simulink library "PAYLOAD_MASTER"  (Simulink 8.8)
settings: Solver=ode45  StartTime=0.0  StopTime=10.0  RelTol=1e-3  EnableMultiTasking=on
libraries: cdsEpicsOut x123, cdsFilt x55, cdsTP x42, cdsFiltCtrl x33, cdsEpicsIn x31, cdsMuxMatrix x17, cdsEpicsBinIn x17, VIS_LIB x13, PAYLOAD_MASTER x13, cdsRms x8, simulink x6, cdsEpicsStringIn x6
(part 12 of 12)

== system PAYLOAD_MASTER/PAYLOADWD/OPLEVAC ==
  TILT_SEG1_In : Inport
  TILT_SEG2_In : Inport  Port=2
  TILT_SEG3_In : Inport  Port=3
  TILT_SEG4_In : Inport  Port=4
  LEN_SEG1_In : Inport  Port=5
  LEN_SEG2_In : Inport  Port=6
  LEN_SEG3_In : Inport  Port=7
  LEN_SEG4_In : Inport  Port=8
  BANDLIM : Subsystem
  LEN_SEG1RMS : cdsRms/Subsystem  Tag=cdsRms  Description=|
      | Purpose:
      | Calculate an RMS based on the input signal.
      settings: AttributesFormatString=%<Tag>
  LEN_SEG1_RMS : cdsTP/Subsystem  Tag=Test Point
      settings: AttributesFormatString=%<Tag>
  LEN_SEG1_RMSMON : cdsEpicsOut/Subsystem  Tag=cdsEpicsOutput  Description=|
      | Purpose:                                          
      | Output a FE signal to an EPICS channel.           
      |                                                   
      | Operation:                                        
      | Takes input value and passes it to EPICS record.  
      |                                                   
      | Usage:                                            
      | Name the part with the desired EPICS rrecord name.
      settings: AttributesFormatString=%<Tag>
  LEN_SEG2RMS : cdsRms/Subsystem  Tag=cdsRms  Description=|
      | Purpose:
      | Calculate an RMS based on the input signal.
      settings: AttributesFormatString=%<Tag>
  LEN_SEG2_RMS : cdsTP/Subsystem  Tag=Test Point
      settings: AttributesFormatString=%<Tag>
  LEN_SEG2_RMSMON : cdsEpicsOut/Subsystem  Tag=cdsEpicsOutput  Description=|
      | Purpose:                                          
      | Output a FE signal to an EPICS channel.           
      |                                                   
      | Operation:                                        
      | Takes input value and passes it to EPICS record.  
      |                                                   
      | Usage:                                            
      | Name the part with the desired EPICS rrecord name.
      settings: AttributesFormatString=%<Tag>
  LEN_SEG3RMS : cdsRms/Subsystem  Tag=cdsRms  Description=|
      | Purpose:
      | Calculate an RMS based on the input signal.
      settings: AttributesFormatString=%<Tag>
  LEN_SEG3_RMS : cdsTP/Subsystem  Tag=Test Point
      settings: AttributesFormatString=%<Tag>
  LEN_SEG3_RMSMON : cdsEpicsOut/Subsystem  Tag=cdsEpicsOutput  Description=|
      | Purpose:                                          
      | Output a FE signal to an EPICS channel.           
      |                                                   
      | Operation:                                        
      | Takes input value and passes it to EPICS record.  
      |                                                   
      | Usage:                                            
      | Name the part with the desired EPICS rrecord name.
      settings: AttributesFormatString=%<Tag>
  LEN_SEG4RMS : cdsRms/Subsystem  Tag=cdsRms  Description=|
      | Purpose:
      | Calculate an RMS based on the input signal.
      settings: AttributesFormatString=%<Tag>
  LEN_SEG4_RMS : cdsTP/Subsystem  Tag=Test Point
      settings: AttributesFormatString=%<Tag>
  LEN_SEG4_RMSMON : cdsEpicsOut/Subsystem  Tag=cdsEpicsOutput  Description=|
      | Purpose:                                          
      | Output a FE signal to an EPICS channel.           
      |                                                   
      | Operation:                                        
      | Takes input value and passes it to EPICS record.  
      |                                                   
      | Usage:                                            
      | Name the part with the desired EPICS rrecord name.
      settings: AttributesFormatString=%<Tag>
  Operator{1,3..8} (7 alike) : RelationalOperator  Operator=>  OutDataTypeStr=boolean  RndMeth=Nearest
  Operator2 : RelationalOperator  Operator=>  OutDataTypeStr=boolean  ZeroCross=off  RndMeth=Nearest
  RMS_MAX : cdsEpicsIn/Subsystem  Tag=cdsEpicsIn  Description=|
      | Purpose:                                                                              
      | Create an EPICS input channel connection to the FE realtime controls.                 
      |                                                                                       
      | Operation:                                                                            
      | Outputs value from an EPICS ai record. Value is floating point with a precision of 3..
      |                                                                                       
      | Usage:                                                                                
      | Name the part with the desired EPICS channel name.
      settings: AttributesFormatString=%<Tag>
  Sum1 : Sum  Inputs=++++++++
  TILT_SEG1RMS : cdsRms/Subsystem  Tag=cdsRms  Description=|
      | Purpose:
      | Calculate an RMS based on the input signal.
      settings: AttributesFormatString=%<Tag>
  TILT_SEG1_RMS : cdsTP/Subsystem  Tag=Test Point
      settings: AttributesFormatString=%<Tag>
  TILT_SEG1_RMSMON : cdsEpicsOut/Subsystem  Tag=cdsEpicsOutput  Description=|
      | Purpose:                                          
      | Output a FE signal to an EPICS channel.           
      |                                                   
      | Operation:                                        
      | Takes input value and passes it to EPICS record.  
      |                                                   
      | Usage:                                            
      | Name the part with the desired EPICS rrecord name.
      settings: AttributesFormatString=%<Tag>
  TILT_SEG2RMS : cdsRms/Subsystem  Tag=cdsRms  Description=|
      | Purpose:
      | Calculate an RMS based on the input signal.
      settings: AttributesFormatString=%<Tag>
  TILT_SEG2_RMS : cdsTP/Subsystem  Tag=Test Point
      settings: AttributesFormatString=%<Tag>
  TILT_SEG2_RMSMON : cdsEpicsOut/Subsystem  Tag=cdsEpicsOutput  Description=|
      | Purpose:                                          
      | Output a FE signal to an EPICS channel.           
      |                                                   
      | Operation:                                        
      | Takes input value and passes it to EPICS record.  
      |                                                   
      | Usage:                                            
      | Name the part with the desired EPICS rrecord name.
      settings: AttributesFormatString=%<Tag>
  TILT_SEG3RMS : cdsRms/Subsystem  Tag=cdsRms  Description=|
      | Purpose:
      | Calculate an RMS based on the input signal.
      settings: AttributesFormatString=%<Tag>
  TILT_SEG3_RMS : cdsTP/Subsystem  Tag=Test Point
      settings: AttributesFormatString=%<Tag>
  TILT_SEG3_RMSMON : cdsEpicsOut/Subsystem  Tag=cdsEpicsOutput  Description=|
      | Purpose:                                          
      | Output a FE signal to an EPICS channel.           
      |                                                   
      | Operation:                                        
      | Takes input value and passes it to EPICS record.  
      |                                                   
      | Usage:                                            
      | Name the part with the desired EPICS rrecord name.
      settings: AttributesFormatString=%<Tag>
  TILT_SEG4RMS : cdsRms/Subsystem  Tag=cdsRms  Description=|
      | Purpose:
      | Calculate an RMS based on the input signal.
      settings: AttributesFormatString=%<Tag>
  TILT_SEG4_RMS : cdsTP/Subsystem  Tag=Test Point
      settings: AttributesFormatString=%<Tag>
  TILT_SEG4_RMSMON : cdsEpicsOut/Subsystem  Tag=cdsEpicsOutput  Description=|
      | Purpose:                                          
      | Output a FE signal to an EPICS channel.           
      |                                                   
      | Operation:                                        
      | Takes input value and passes it to EPICS record.  
      |                                                   
      | Usage:                                            
      | Name the part with the desired EPICS rrecord name.
      settings: AttributesFormatString=%<Tag>
  FLAG : Outport
  wires:
  TILT_SEG3_RMSMON/1 -> Operator3/1
  TILT_SEG2_RMSMON/1 -> Operator2/1
  TILT_SEG1_RMSMON/1 -> Operator1/1
  Sum1/1 -> FLAG/1
  TILT_SEG3RMS/1 -> TILT_SEG3_RMSMON/1, TILT_SEG3_RMS/1
  TILT_SEG1RMS/1 -> TILT_SEG1_RMSMON/1, TILT_SEG1_RMS/1
  TILT_SEG2RMS/1 -> TILT_SEG2_RMSMON/1, TILT_SEG2_RMS/1
  Operator3/1 -> Sum1/3
  Operator2/1 -> Sum1/2
  Operator1/1 -> Sum1/1
  TILT_SEG1_In/1 -> BANDLIM/1(TILT_SEG1_In)
  TILT_SEG2_In/1 -> BANDLIM/2(TILT_SEG2_In)
  TILT_SEG3_In/1 -> BANDLIM/3(TILT_SEG3_In)
  BANDLIM/1(TILT_SEG1_Out) -> TILT_SEG1RMS/1
  BANDLIM/2(TILT_SEG2_Out) -> TILT_SEG2RMS/1
  BANDLIM/3(TILT_SEG3_Out) -> TILT_SEG3RMS/1
  TILT_SEG4_In/1 -> BANDLIM/4(TILT_SEG4_In)
  LEN_SEG1_In/1 -> BANDLIM/5(LEN_SEG1_In)
  LEN_SEG2_In/1 -> BANDLIM/6(LEN_SEG2_In)
  LEN_SEG3_In/1 -> BANDLIM/7(LEN_SEG3_In)
  LEN_SEG4_In/1 -> BANDLIM/8(LEN_SEG4_In)
  TILT_SEG4RMS/1 -> TILT_SEG4_RMSMON/1, TILT_SEG4_RMS/1
  LEN_SEG1RMS/1 -> LEN_SEG1_RMSMON/1, LEN_SEG1_RMS/1
  LEN_SEG2RMS/1 -> LEN_SEG2_RMSMON/1, LEN_SEG2_RMS/1
  LEN_SEG3RMS/1 -> LEN_SEG3_RMSMON/1, LEN_SEG3_RMS/1
  LEN_SEG4RMS/1 -> LEN_SEG4_RMSMON/1, LEN_SEG4_RMS/1
  BANDLIM/4(TILT_SEG4_Out) -> TILT_SEG4RMS/1
  BANDLIM/5(LEN_SEG1_Out) -> LEN_SEG1RMS/1
  BANDLIM/6(LEN_SEG2_Out) -> LEN_SEG2RMS/1
  BANDLIM/7(LEN_SEG3_Out) -> LEN_SEG3RMS/1
  BANDLIM/8(LEN_SEG4_Out) -> LEN_SEG4RMS/1
  TILT_SEG4_RMSMON/1 -> Operator4/1
  LEN_SEG1_RMSMON/1 -> Operator5/1
  LEN_SEG2_RMSMON/1 -> Operator7/1
  LEN_SEG3_RMSMON/1 -> Operator6/1
  LEN_SEG4_RMSMON/1 -> Operator8/1
  RMS_MAX/1 -> Operator8/2, Operator6/2, Operator7/2, Operator5/2, Operator4/2, Operator3/2, Operator2/2, Operator1/2
  Operator4/1 -> Sum1/4
  Operator5/1 -> Sum1/5
  Operator7/1 -> Sum1/6
  Operator6/1 -> Sum1/7
  Operator8/1 -> Sum1/8

== system PAYLOAD_MASTER/PAYLOAD_MASTER/BIO ==
  note: 12 Bit Word
  note: 12 Bit Word
  TM_ISC_CTRL : Inport
  TM_MON_In : Inport  Port=2
  IM1_CTRL : Inport  Port=3
  IM1_MON_In : Inport  Port=4
  IM2_ISC_CTRL : Inport  Port=5
  IM2_MON_In : Inport  Port=6
  IM1 : STATE_BIO_MASTER/UIM_BIO_MASTER
  IM2 : STATE_BIO_MASTER/UIM_BIO_MASTER
  TM : STATE_BIO_MASTER/UIM_BIO_MASTER
  TM_BO_CTRL_Out : Outport
  TM_MASK_Out : Outport  Port=2
  TM_CTRL_Out : Outport  Port=3
  IM1_BO_CTRL_Out : Outport  Port=4
  IM1_MASK_Out : Outport  Port=5
  IM1_CTRL_Out : Outport  Port=6
  IM2_BO_CTRL_Out : Outport  Port=7
  IM2_MASK_Out : Outport  Port=8
  IM2_CTRL_Out : Outport  Port=9
  wires:
  IM2/3 -> IM2_BO_CTRL_Out/1
  IM2/2 -> IM2_CTRL_Out/1
  IM2/1 -> IM2_MASK_Out/1
  IM1/3 -> IM1_BO_CTRL_Out/1
  IM1/2 -> IM1_CTRL_Out/1
  IM1/1 -> IM1_MASK_Out/1
  TM/3 -> TM_BO_CTRL_Out/1
  TM/2 -> TM_CTRL_Out/1
  TM/1 -> TM_MASK_Out/1
  IM2_ISC_CTRL/1 -> IM2/1
  IM2_MON_In/1 -> IM2/2
  IM1_MON_In/1 -> IM1/2
  IM1_CTRL/1 -> IM1/1
  TM_ISC_CTRL/1 -> TM/1
  TM_MON_In/1 -> TM/2

== system PAYLOAD_MASTER/PAYLOADWD/OPLEVAC/BANDLIM ==
  TILT_SEG1_In : Inport
  TILT_SEG2_In : Inport  Port=2
  TILT_SEG3_In : Inport  Port=3
  TILT_SEG4_In : Inport  Port=4
  LEN_SEG1_In : Inport  Port=5
  LEN_SEG2_In : Inport  Port=6
  LEN_SEG3_In : Inport  Port=7
  LEN_SEG4_In : Inport  Port=8
  LEN_SEG1 : cdsFilt/Subsystem  Tag=cdsFilt  Description=|
      | Purpose:                                                                                                                                                                                                                                  
      | Standard CDS IIR filter module.                                                                                                                                                                                                           
      |                                                                                                                                                                                                                                           
      | Operation:                                                                                                                                                                                                                                
      | Consists of 10 second order section IIR filters, plus a ramped gain stage. In FE code, also provides pre-defined test points and excitation channel inputs. The filter coefficients are defined in the LIGO system using the 'foton' tool.
      |                                                                                                                                                                                                                                           
      | Usage:                                                                                                                                                                                                                                    
      | Name the part with the desired filter module name.
      settings: AttributesFormatString=%<Tag>
  LEN_SEG2 : cdsFilt/Subsystem  Tag=cdsFilt  Description=|
      | Purpose:                                                                                                                                                                                                                                  
      | Standard CDS IIR filter module.                                                                                                                                                                                                           
      |                                                                                                                                                                                                                                           
      | Operation:                                                                                                                                                                                                                                
      | Consists of 10 second order section IIR filters, plus a ramped gain stage. In FE code, also provides pre-defined test points and excitation channel inputs. The filter coefficients are defined in the LIGO system using the 'foton' tool.
      |                                                                                                                                                                                                                                           
      | Usage:                                                                                                                                                                                                                                    
      | Name the part with the desired filter module name.
      settings: AttributesFormatString=%<Tag>
  LEN_SEG3 : cdsFilt/Subsystem  Tag=cdsFilt  Description=|
      | Purpose:                                                                                                                                                                                                                                  
      | Standard CDS IIR filter module.                                                                                                                                                                                                           
      |                                                                                                                                                                                                                                           
      | Operation:                                                                                                                                                                                                                                
      | Consists of 10 second order section IIR filters, plus a ramped gain stage. In FE code, also provides pre-defined test points and excitation channel inputs. The filter coefficients are defined in the LIGO system using the 'foton' tool.
      |                                                                                                                                                                                                                                           
      | Usage:                                                                                                                                                                                                                                    
      | Name the part with the desired filter module name.
      settings: AttributesFormatString=%<Tag>
  LEN_SEG4 : cdsFilt/Subsystem  Tag=cdsFilt  Description=|
      | Purpose:                                                                                                                                                                                                                                  
      | Standard CDS IIR filter module.                                                                                                                                                                                                           
      |                                                                                                                                                                                                                                           
      | Operation:                                                                                                                                                                                                                                
      | Consists of 10 second order section IIR filters, plus a ramped gain stage. In FE code, also provides pre-defined test points and excitation channel inputs. The filter coefficients are defined in the LIGO system using the 'foton' tool.
      |                                                                                                                                                                                                                                           
      | Usage:                                                                                                                                                                                                                                    
      | Name the part with the desired filter module name.
      settings: AttributesFormatString=%<Tag>
  TILT_SEG1 : cdsFilt/Subsystem  Tag=cdsFilt  Description=|
      | Purpose:                                                                                                                                                                                                                                  
      | Standard CDS IIR filter module.                                                                                                                                                                                                           
      |                                                                                                                                                                                                                                           
      | Operation:                                                                                                                                                                                                                                
      | Consists of 10 second order section IIR filters, plus a ramped gain stage. In FE code, also provides pre-defined test points and excitation channel inputs. The filter coefficients are defined in the LIGO system using the 'foton' tool.
      |                                                                                                                                                                                                                                           
      | Usage:                                                                                                                                                                                                                                    
      | Name the part with the desired filter module name.
      settings: AttributesFormatString=%<Tag>
  TILT_SEG2 : cdsFilt/Subsystem  Tag=cdsFilt  Description=|
      | Purpose:                                                                                                                                                                                                                                  
      | Standard CDS IIR filter module.                                                                                                                                                                                                           
      |                                                                                                                                                                                                                                           
      | Operation:                                                                                                                                                                                                                                
      | Consists of 10 second order section IIR filters, plus a ramped gain stage. In FE code, also provides pre-defined test points and excitation channel inputs. The filter coefficients are defined in the LIGO system using the 'foton' tool.
      |                                                                                                                                                                                                                                           
      | Usage:                                                                                                                                                                                                                                    
      | Name the part with the desired filter module name.
      settings: AttributesFormatString=%<Tag>
  TILT_SEG3 : cdsFilt/Subsystem  Tag=cdsFilt  Description=|
      | Purpose:                                                                                                                                                                                                                                  
      | Standard CDS IIR filter module.                                                                                                                                                                                                           
      |                                                                                                                                                                                                                                           
      | Operation:                                                                                                                                                                                                                                
      | Consists of 10 second order section IIR filters, plus a ramped gain stage. In FE code, also provides pre-defined test points and excitation channel inputs. The filter coefficients are defined in the LIGO system using the 'foton' tool.
      |                                                                                                                                                                                                                                           
      | Usage:                                                                                                                                                                                                                                    
      | Name the part with the desired filter module name.
      settings: AttributesFormatString=%<Tag>
  TILT_SEG4 : cdsFilt/Subsystem  Tag=cdsFilt  Description=|
      | Purpose:                                                                                                                                                                                                                                  
      | Standard CDS IIR filter module.                                                                                                                                                                                                           
      |                                                                                                                                                                                                                                           
      | Operation:                                                                                                                                                                                                                                
      | Consists of 10 second order section IIR filters, plus a ramped gain stage. In FE code, also provides pre-defined test points and excitation channel inputs. The filter coefficients are defined in the LIGO system using the 'foton' tool.
      |                                                                                                                                                                                                                                           
      | Usage:                                                                                                                                                                                                                                    
      | Name the part with the desired filter module name.
      settings: AttributesFormatString=%<Tag>
  TILT_SEG1_Out : Outport
  TILT_SEG2_Out : Outport  Port=2
  TILT_SEG3_Out : Outport  Port=3
  TILT_SEG4_Out : Outport  Port=4
  LEN_SEG1_Out : Outport  Port=5
  LEN_SEG2_Out : Outport  Port=6
  LEN_SEG3_Out : Outport  Port=7
  LEN_SEG4_Out : Outport  Port=8
  wires:
  TILT_SEG2_In/1 -> TILT_SEG2/1
  TILT_SEG1_In/1 -> TILT_SEG1/1
  TILT_SEG2/1 -> TILT_SEG2_Out/1
  TILT_SEG1/1 -> TILT_SEG1_Out/1
  TILT_SEG4_In/1 -> TILT_SEG4/1
  TILT_SEG3_In/1 -> TILT_SEG3/1
  TILT_SEG4/1 -> TILT_SEG4_Out/1
  TILT_SEG3/1 -> TILT_SEG3_Out/1
  LEN_SEG1_In/1 -> LEN_SEG1/1
  LEN_SEG1/1 -> LEN_SEG1_Out/1
  LEN_SEG2_In/1 -> LEN_SEG2/1
  LEN_SEG2/1 -> LEN_SEG2_Out/1
  LEN_SEG3_In/1 -> LEN_SEG3/1
  LEN_SEG3/1 -> LEN_SEG3_Out/1
  LEN_SEG4_In/1 -> LEN_SEG4/1
  LEN_SEG4/1 -> LEN_SEG4_Out/1
